simulink subsystem "Resonant_load"  (R2024b)
settings: Solver=VariableStepAuto  StartTime=0.0  StopTime=10.0  RelTol=1e-3
undefined symbols (not defined in the file or in its folder): mld
settings Model: Creator=Federico Bergami  LastModifiedBy=Federico Bergami

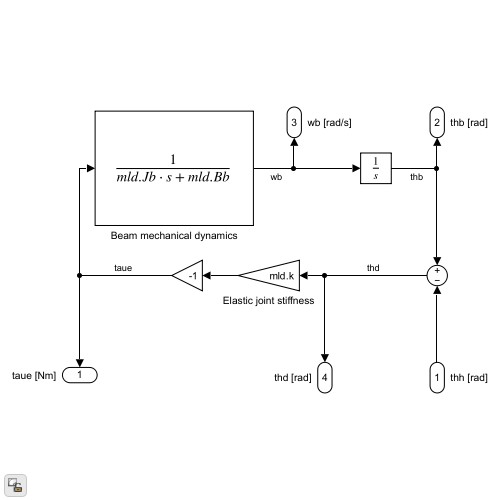
[thumbnail: Simulink's stored preview of the top-level diagram]
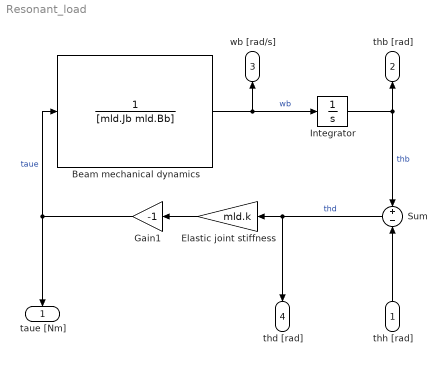
== system Resonant_load ==
  thh [rad] : Inport
  Beam mechanical dynamics : TransferFcn  Denominator=[mld.Jb mld.Bb]
  Elastic joint stiffness : Gain  Gain=mld.k
  Gain1 : Gain  Gain=-1
  Integrator : Integrator  ZeroCross=off
  Sum : Sum  Inputs=+|-
  taue [Nm] : Outport
  thb [rad] : Outport  Port=2
  wb [rad/s] : Outport  Port=3
  thd [rad] : Outport  Port=4
  wires:
  Elastic joint stiffness/1 -> Gain1/1
  Sum/1 -> thd [rad]/1, Elastic joint stiffness/1  "thd"
  Integrator/1 -> Sum/1, thb [rad]/1  "thb"
  thh [rad]/1 -> Sum/2
  Gain1/1 -> Beam mechanical dynamics/1, taue [Nm]/1  "taue"
  Beam mechanical dynamics/1 -> wb [rad/s]/1, Integrator/1  "wb"
